simulink model "Pioneer_sim_ucla_mae154S_post"  (Simulink 8.5)
settings: Solver=ode45  StartTime=0.0  StopTime=10000  RelTol=1e-3
model workspace (MATLAB code in the model file):
  | init_dynamics;
values from neighbouring files (symbols this model uses):
  bw = 16.90    (= 16.9)    [get_coeffs.m]    (also in get_coeffs_from_optimization.m; init_dynamics.m)
  cbar = 1.80    (= 1.8)    [get_coeffs.m]    (also in get_coeffs_from_optimization.m; init_dynamics.m)
  grav = 32.17405    [aero_dyn.m]    (also in init_dynamics.m)
  rho = 0.002379    [init_dynamics.m]
  Sw = 30.42    [init_dynamics.m]
  thrust_bx = 89.8    [init_dynamics.m]
libraries: simulink x3
settings Model: Creator=jwm26790  LastModifiedBy=matsuka
settings OptimizationCC: InitFltsAndDblsToZero=on
settings DebuggingCC: SaveWithParameterizedLinksMsg=none  SolverPrmCheckMsg=warning  FcnCallInpInsideContextMsg=UseLocalSettings
settings GRTTargetCC: TargetFcnLib=ansi_tfl_tmw.mat

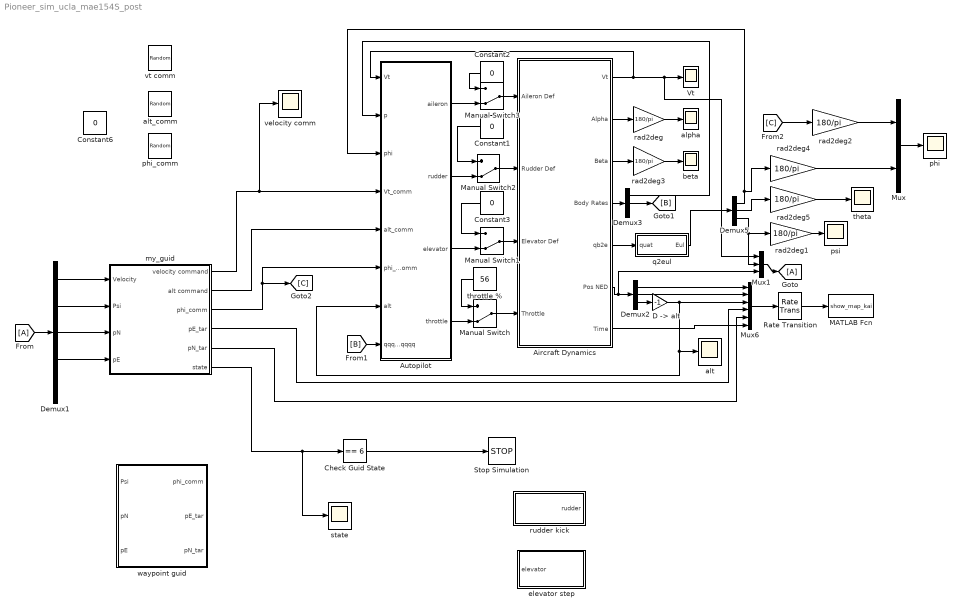
== system Pioneer_sim_ucla_mae154S_post ==
  Aircraft Dynamics : Subsystem
  Autopilot : Subsystem
  Check Guid State : simulink/Logic and Bit Operations/Compare To Constant  relop===  const=6  OutDataTypeStr=boolean
  Constant{1..3,6} (4 alike) : Constant  Value=0
  "D -> alt" : Gain  Gain=-1
  Demux1 : Demux  Outputs=5
  Demux2 : Demux  Outputs=3
  Demux3 : Demux  Outputs=3
  Demux5 : Demux  Outputs=3
  MATLAB Fcn : MATLABFcn  MATLABFcn=show_map_kai  OutputDimensions=0
  Manual Switch{,1..3} (4 alike) : ManualSwitch  CurrentSetting=0
  Mux : Mux  Inputs=2
  Mux1 : Mux  Inputs=[1 1 3]
  Mux6 : Mux  Inputs=6
  Rate Transition : RateTransition  OutPortSampleTime=10
  Stop Simulation : Stop
  Vt : Scope
      settings: TimeRange=50  YMin=131.75  YMax=132.6  SaveName=ScopeData8
  alpha : Scope
      settings: TimeRange=50  YMin=6.9  YMax=7.9
  alt : Scope
      settings: TimeRange=50  YMin=999.5  YMax=1004.5  SaveName=ScopeData14
  alt_comm : UniformRandomNumber  Minimum=1000  Maximum=1500  Seed=2  SampleTime=50
  beta : Scope
      settings: TimeRange=200  YMin=-4  YMax=3  SaveName=ScopeData4
  elevator step : Subsystem
  my_guid : Subsystem
  phi : Scope
      settings: TimeRange=50  YMin=-30  YMax=40  SaveName=ScopeData7
  phi_comm : UniformRandomNumber  Minimum=-.5  Maximum=.5  Seed=3  SampleTime=20
  psi : Scope
      settings: TimeRange=100  YMin=-172.5  YMax=-130  SaveName=ScopeData9
  q2eul : Subsystem
  rad2deg{,1..5} (6 alike) : Gain  Gain=180/pi
  rudder kick : Subsystem
  state : Scope
      settings: TimeRange=50  YMin=2  YMax=2  SaveName=ScopeData15
  theta : Scope
      settings: TimeRange=50  YMin=5.5  YMax=9
  throttle % : Constant  Value=56
  velocity comm : Scope
      settings: TimeRange=50  YMin=100  YMax=100  SaveName=ScopeData16
  vt comm : UniformRandomNumber  Minimum=100  Maximum=130  Seed=2  SampleTime=20
  waypoint guid : Subsystem
  wires:
  Aircraft Dynamics/5(qb2e) -> q2eul/1(quat)
  Aircraft Dynamics/4(Body Rates) -> Demux3/1
  Aircraft Dynamics/1(Vt) -> Autopilot/1(Vt), Vt/1, Mux1/1
  Aircraft Dynamics/6(Pos NED) -> Demux2/1, Mux1/3
  Demux2/3 -> "D -> alt"/1
  "D -> alt"/1 -> Mux6/3, alt/1, Autopilot/7(alt)
  Aircraft Dynamics/2(Alpha) -> rad2deg/1
  rad2deg/1 -> alpha/1
  Aircraft Dynamics/3(Beta) -> rad2deg3/1
  rad2deg3/1 -> beta/1
  q2eul/1(Eul) -> Demux5/1
  Demux5/1 -> Autopilot/3(phi), rad2deg4/1
  Demux3/1 -> Autopilot/2(p)
  Demux2/1 -> Mux6/1
  Demux2/2 -> Mux6/2
  rad2deg1/1 -> psi/1
  rad2deg4/1 -> Mux/2
  rad2deg5/1 -> theta/1
  Demux5/3 -> rad2deg1/1, Mux1/2
  Demux5/2 -> rad2deg5/1
  my_guid/4(pE_tar) -> Mux6/4
  my_guid/5(pN_tar) -> Mux6/5
  Mux1/1 -> [A]
  [A] -> Demux1/1
  Rate Transition/1 -> MATLAB Fcn/1
  Mux6/1 -> Rate Transition/1
  Manual Switch/1 -> Aircraft Dynamics/4(Throttle)
  Manual Switch1/1 -> Aircraft Dynamics/3(Elevator Def)
  throttle %/1 -> Manual Switch/1
  Autopilot/4(throttle) -> Manual Switch/2
  Autopilot/3(elevator) -> Manual Switch1/2
  Manual Switch2/1 -> Aircraft Dynamics/2(Rudder Def)
  Autopilot/2(rudder) -> Manual Switch2/2
  Manual Switch3/1 -> Aircraft Dynamics/1(Aileron Def)
  Autopilot/1(aileron) -> Manual Switch3/2
  Constant2/1 -> Manual Switch3/1
  my_guid/2(alt command) -> Autopilot/5(alt_comm)
  Constant3/1 -> Manual Switch1/1
  Constant1/1 -> Manual Switch2/1
  Demux3/2 -> [B]
  [B] -> Autopilot/8(qqqqqqqqqqqqqqqqqqqqqqqqqqqqqqqqqqqqqqqqqqqqqqqqqqqqqqqqqqqqqqqqqqqqqqqqqqqqqqqqqqqqqqqqqqqqqq)
  my_guid/3(phi_comm) -> Autopilot/6(phi_comm), [C]
  my_guid/1(velocity command) -> velocity comm/1, Autopilot/4(Vt_comm)
  Aircraft Dynamics/7(Time) -> Mux6/6
  Demux1/2 -> my_guid/2(Psi)
  Demux1/3 -> my_guid/3(pN)
  Demux1/4 -> my_guid/4(pE)
  Demux1/1 -> my_guid/1(Velocity)
  [C] -> rad2deg2/1
  Mux/1 -> phi/1
  rad2deg2/1 -> Mux/1
  my_guid/6(state) -> state/1, Check Guid State/1
  Check Guid State/1 -> Stop Simulation/1

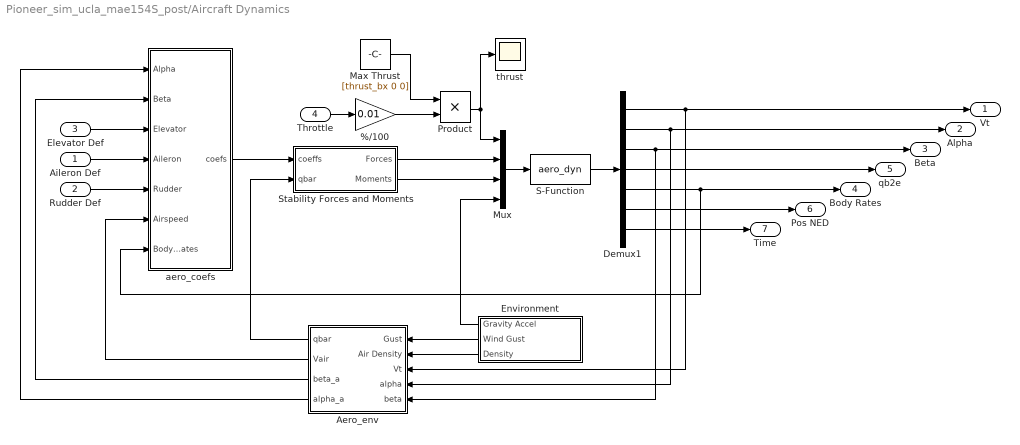
== system Pioneer_sim_ucla_mae154S_post/Aircraft Dynamics ==
  Aileron Def : Inport
  Rudder Def : Inport  Port=2
  Elevator Def : Inport  Port=3
  Throttle : Inport  Port=4
  %/100 : Gain  Gain=0.01
  Aero_env : Subsystem
  Demux1 : Demux  Outputs=[1 1 1 4 3 3 1]
  Environment : Subsystem
  Max Thrust : Constant  Value=[thrust_bx 0 0]
  Mux : Mux
  Product : Product  RndMeth=Zero
  S-Function : S-Function  FunctionName=aero_dyn
  Stability Forces and Moments : Subsystem
  aero_coefs : Subsystem
  thrust : Scope
      settings: YMin=0  YMax=90  SaveName=ScopeData6
  Vt : Outport
  Alpha : Outport  Port=2
  Beta : Outport  Port=3
  Body Rates : Outport  Port=4
  qb2e : Outport  Port=5
  Pos NED : Outport  Port=6
  Time : Outport  Port=7
  wires:
  Demux1/7 -> Time/1
  Demux1/3 -> Aero_env/5(beta), Beta/1
  Demux1/2 -> Aero_env/4(alpha), Alpha/1
  Demux1/1 -> Aero_env/3(Vt), Vt/1
  S-Function/1 -> Demux1/1
  Mux/1 -> S-Function/1
  Demux1/4 -> qb2e/1
  Environment/1(Gravity Accel) -> Mux/4
  Rudder Def/1 -> aero_coefs/5(Rudder)
  Aileron Def/1 -> aero_coefs/4(Aileron)
  Demux1/6 -> Pos NED/1
  Demux1/5 -> aero_coefs/7(Body Rates), Body Rates/1
  Aero_env/2(Vair) -> aero_coefs/6(Airspeed)
  Aero_env/1(qbar) -> Stability Forces and Moments/2(qbar)
  Aero_env/3(beta_a) -> aero_coefs/2(Beta)
  Aero_env/4(alpha_a) -> aero_coefs/1(Alpha)
  Environment/2(Wind Gust) -> Aero_env/1(Gust)
  Environment/3(Density) -> Aero_env/2(Air Density)
  Stability Forces and Moments/1(Forces) -> Mux/2
  aero_coefs/1(coefs) -> Stability Forces and Moments/1(coeffs)
  Stability Forces and Moments/2(Moments) -> Mux/3
  Elevator Def/1 -> aero_coefs/3(Elevator)
  Product/1 -> Mux/1, thrust/1
  Max Thrust/1 -> Product/1
  Throttle/1 -> %/100/1
  %/100/1 -> Product/2

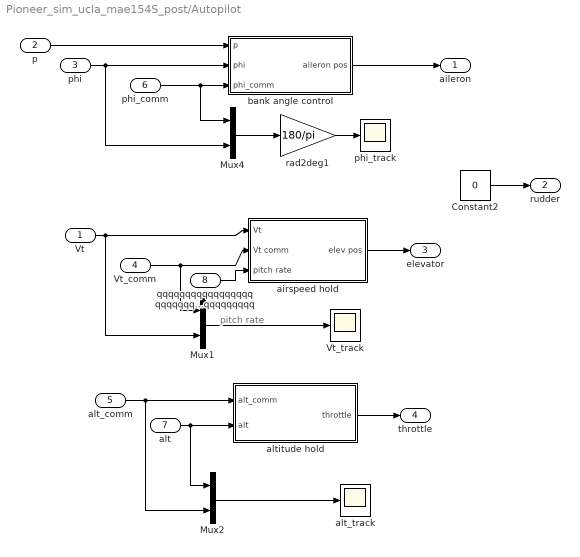
== system Pioneer_sim_ucla_mae154S_post/Autopilot ==
  note: pitch rate
  Vt : Inport
  p : Inport  Port=2
  phi : Inport  Port=3
  Vt_comm : Inport  Port=4
  alt_comm : Inport  Port=5
  phi_comm : Inport  Port=6
  alt : Inport  Port=7
  qqqqqqqqqqqqqqqqqqqqqqqqqqqqqqqqqqqqqqqqqqqqqqqqqqqqqqqqqqqqqqqqqqqqqqqqqqqqqqqqqqqqqqqqqqqqqq : Inport  Port=8
  Constant2 : Constant  Value=0
  Mux1 : Mux  Inputs=2
  Mux2 : Mux  Inputs=2
  Mux4 : Mux  Inputs=2
  Vt_track : Scope
      settings: TimeRange=60  YMin=90  YMax=135  SaveName=ScopeData11
  airspeed hold : Subsystem
  alt_track : Scope
      settings: TimeRange=200  YMin=900  YMax=1600  SaveName=ScopeData12
  altitude hold : Subsystem
  bank angle control : Subsystem
  phi_track : Scope
      settings: TimeRange=200  YMin=-35  YMax=35  SaveName=ScopeData5
  rad2deg1 : Gain  Gain=180/pi
  aileron : Outport
  rudder : Outport  Port=2
  elevator : Outport  Port=3
  throttle : Outport  Port=4
  wires:
  altitude hold/1(throttle) -> throttle/1
  airspeed hold/1(elev pos) -> elevator/1
  bank angle control/1(aileron pos) -> aileron/1
  p/1 -> bank angle control/1(p)
  phi/1 -> bank angle control/2(phi), Mux4/2
  Vt/1 -> airspeed hold/1(Vt), Mux1/2
  alt/1 -> altitude hold/2(alt), Mux2/1
  Mux4/1 -> rad2deg1/1
  rad2deg1/1 -> phi_track/1
  Mux1/1 -> Vt_track/1
  Mux2/1 -> alt_track/1
  alt_comm/1 -> altitude hold/1(alt_comm), Mux2/2
  Vt_comm/1 -> airspeed hold/2(Vt comm), Mux1/1
  phi_comm/1 -> bank angle control/3(phi_comm), Mux4/1
  Constant2/1 -> rudder/1
  qqqqqqqqqqqqqqqqqqqqqqqqqqqqqqqqqqqqqqqqqqqqqqqqqqqqqqqqqqqqqqqqqqqqqqqqqqqqqqqqqqqqqqqqqqqqqq/1 -> airspeed hold/3(pitch rate)

== system Pioneer_sim_ucla_mae154S_post/elevator step ==
  Step4 : Step  Time=5  After=-2*pi/180  SampleTime=0
  Step5 : Step  Time=10  After=10*pi/180  SampleTime=0
  Sum1 : Sum  SaturateOnIntegerOverflow=on
  actuator lag : TransferFcn  Numerator=[10]  Denominator=[1 10]
  elevator1 : Scope
      settings: TimeRange=50  YMin=0  YMax=12  SaveName=ScopeData13
  rad2deg2 : Gain  Gain=180/pi
  elevator : Outport
  wires:
  Step4/1 -> Sum1/1
  rad2deg2/1 -> elevator1/1
  actuator lag/1 -> elevator/1, rad2deg2/1
  Sum1/1 -> actuator lag/1

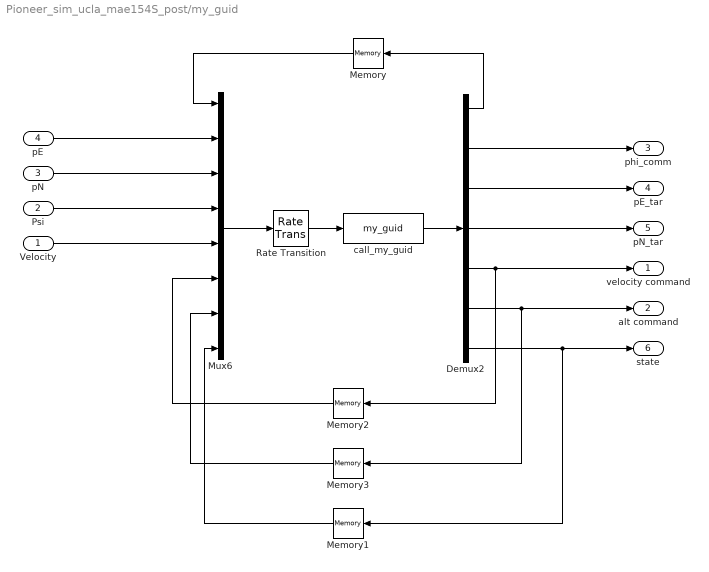
== system Pioneer_sim_ucla_mae154S_post/my_guid ==
  Velocity : Inport
  Psi : Inport  Port=2
  pN : Inport  Port=3
  pE : Inport  Port=4
  Demux2 : Demux  Outputs=7
  Memory : Memory  X0=1
  Memory1 : Memory
  Memory2 : Memory  X0=118.1
  Memory3 : Memory  X0=100
  Mux6 : Mux  Inputs=8
  Rate Transition : RateTransition  OutPortSampleTime=0.1
  call_my_guid : MATLABFcn  MATLABFcn=my_guid  OutputDimensions=7  SampleTime=.5
  velocity command : Outport
  alt command : Outport  Port=2
  phi_comm : Outport  Port=3
  pE_tar : Outport  Port=4
  pN_tar : Outport  Port=5
  state : Outport  Port=6
  wires:
  call_my_guid/1 -> Demux2/1
  Demux2/2 -> phi_comm/1
  Demux2/3 -> pE_tar/1
  Demux2/4 -> pN_tar/1
  pE/1 -> Mux6/2
  pN/1 -> Mux6/3
  Psi/1 -> Mux6/4
  Memory/1 -> Mux6/1
  Rate Transition/1 -> call_my_guid/1
  Mux6/1 -> Rate Transition/1
  Demux2/1 -> Memory/1
  Velocity/1 -> Mux6/5
  Demux2/5 -> Memory2/1, velocity command/1
  Memory1/1 -> Mux6/8
  Memory2/1 -> Mux6/6
  Demux2/7 -> Memory1/1, state/1
  Demux2/6 -> Memory3/1, alt command/1
  Memory3/1 -> Mux6/7

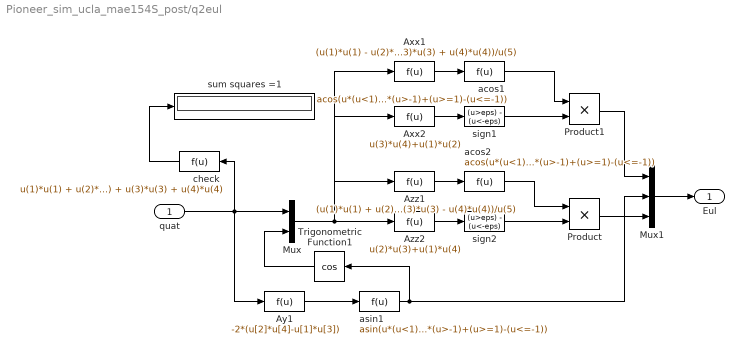
== system Pioneer_sim_ucla_mae154S_post/q2eul ==
  quat : Inport
  Axx1 : Fcn  Expr=(u(1)*u(1) - u(2)*u(2) - u(3)*u(3) + u(4)*u(4))/u(5)
  Axx2 : Fcn  Expr=u(3)*u(4)+u(1)*u(2)
  Ay1 : Fcn  Expr=-2*(u[2]*u[4]-u[1]*u[3])
  Azz1 : Fcn  Expr=(u(1)*u(1) + u(2)*u(2) - u(3)*u(3) - u(4)*u(4))/u(5)
  Azz2 : Fcn  Expr=u(2)*u(3)+u(1)*u(4)
  Mux : Mux  Inputs=2
  Mux1 : Mux  Inputs=3
  Product : Product  SaturateOnIntegerOverflow=on  RndMeth=Zero  InputSameDT=on  OutDataTypeStr=Inherit: Same as first input
  Product1 : Product  SaturateOnIntegerOverflow=on  RndMeth=Zero  InputSameDT=on  OutDataTypeStr=Inherit: Same as first input
  Trigonometric Function1 : Trigonometry  Operator=cos
  acos1 : Fcn  Expr=acos(u*(u<1)*(u>-1)+(u>=1)-(u<=-1))
  acos2 : Fcn  Expr=acos(u*(u<1)*(u>-1)+(u>=1)-(u<=-1))
  "asin1 " : Fcn  Expr=asin(u*(u<1)*(u>-1)+(u>=1)-(u<=-1))
  check : Fcn  Expr=u(1)*u(1) + u(2)*u(2) + u(3)*u(3) + u(4)*u(4)
  sign1 : Fcn  Expr=(u>eps) - (u<-eps)
  sign2 : Fcn  Expr=(u>eps) - (u<-eps)
  sum squares =1 : Display
      settings: Format=long_e
  Eul : Outport  InitialOutput=0
  wires:
  sign1/1 -> Product1/2
  Mux/1 -> Azz2/1, Axx2/1, Azz1/1, Axx1/1
  Trigonometric Function1/1 -> Mux/2
  Ay1/1 -> "asin1 "/1
  Product/1 -> Mux1/3
  acos2/1 -> Product/1
  Product1/1 -> Mux1/1
  acos1/1 -> Product1/1
  sign2/1 -> Product/2
  Axx2/1 -> sign1/1
  Azz1/1 -> acos2/1
  Azz2/1 -> sign2/1
  Axx1/1 -> acos1/1
  "asin1 "/1 -> Mux1/2, Trigonometric Function1/1
  quat/1 -> Mux/1, check/1, Ay1/1
  check/1 -> sum squares =1/1
  Mux1/1 -> Eul/1

== system Pioneer_sim_ucla_mae154S_post/rudder kick ==
  note: rudder kick
  Step1 : Step  Time=10  After=10*pi/180  SampleTime=0
  Step2 : Step  Time=10.5  After=-20*pi/180  SampleTime=0
  Step3 : Step  Time=11  After=10*pi/180  SampleTime=0
  Sum2 : Sum  Inputs=+++  SaturateOnIntegerOverflow=on
  actuator lag : TransferFcn  Numerator=[10]  Denominator=[1 10]
  rad2deg2 : Gain  Gain=180/pi
  rudder1 : Scope
      settings: TimeRange=50  YMin=0  YMax=12  SaveName=ScopeData2
  rudder : Outport
  wires:
  Step1/1 -> Sum2/1
  Step2/1 -> Sum2/2
  Step3/1 -> Sum2/3
  Sum2/1 -> actuator lag/1
  rad2deg2/1 -> rudder1/1
  actuator lag/1 -> rudder/1, rad2deg2/1

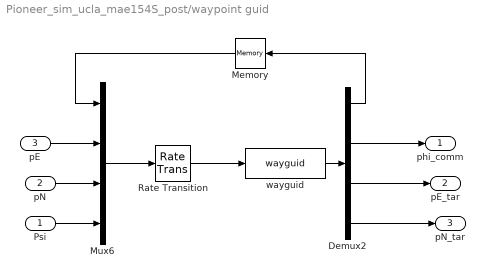
== system Pioneer_sim_ucla_mae154S_post/waypoint guid ==
  Psi : Inport
  pN : Inport  Port=2
  pE : Inport  Port=3
  Demux2 : Demux
  Memory : Memory
  Mux6 : Mux
  Rate Transition : RateTransition  OutPortSampleTime=0.5
  wayguid : MATLABFcn  MATLABFcn=wayguid  OutputDimensions=4  SampleTime=.5
  phi_comm : Outport
  pE_tar : Outport  Port=2
  pN_tar : Outport  Port=3
  wires:
  wayguid/1 -> Demux2/1
  Demux2/2 -> phi_comm/1
  Demux2/3 -> pE_tar/1
  Demux2/4 -> pN_tar/1
  pE/1 -> Mux6/2
  pN/1 -> Mux6/3
  Psi/1 -> Mux6/4
  Memory/1 -> Mux6/1
  Rate Transition/1 -> wayguid/1
  Mux6/1 -> Rate Transition/1
  Demux2/1 -> Memory/1

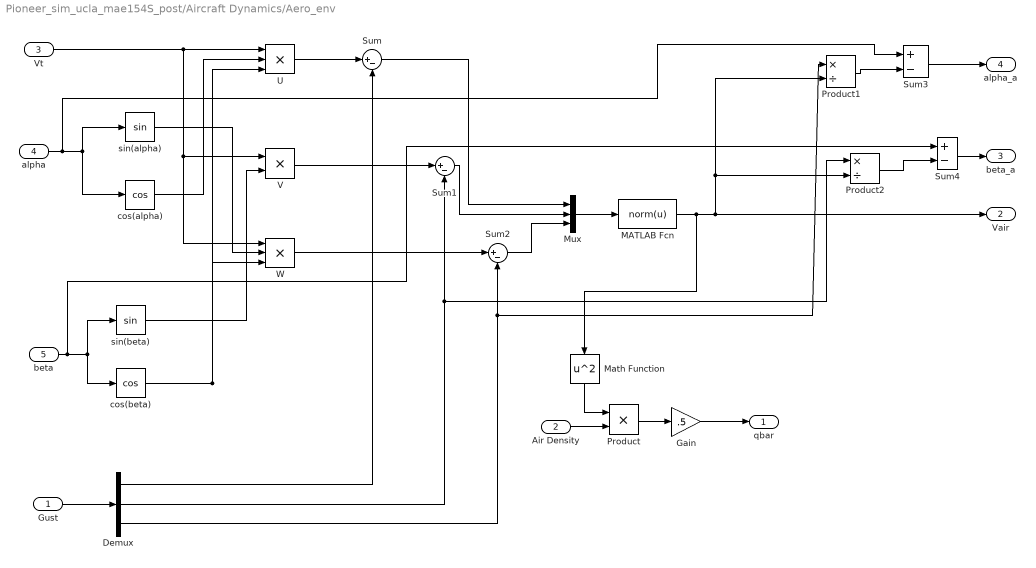
== system Pioneer_sim_ucla_mae154S_post/Aircraft Dynamics/Aero_env ==
  Gust : Inport
  Air Density : Inport  Port=2
  Vt : Inport  Port=3
  alpha : Inport  Port=4
  beta : Inport  Port=5
  Demux : Demux  Outputs=3
  Gain : Gain  Gain=.5
  MATLAB Fcn : MATLABFcn  MATLABFcn=norm(u)
  Math Function : Math  Operator=square  SaturateOnIntegerOverflow=on
  Mux : Mux  Inputs=3
  Product : Product  RndMeth=Zero
  Product1 : Product  Inputs=*/  RndMeth=Zero
  Product2 : Product  Inputs=*/  RndMeth=Zero
  Sum : Sum  Inputs=|+-
  Sum1 : Sum  Inputs=|+-
  Sum2 : Sum  Inputs=|+-
  Sum3 : Sum  Inputs=+-
  Sum4 : Sum  Inputs=+-
  U : Product  Inputs=3
  V : Product
  W : Product  Inputs=3
  cos(alpha) : Trigonometry  Operator=cos
  cos(beta) : Trigonometry  Operator=cos
  sin(alpha) : Trigonometry
  sin(beta) : Trigonometry
  qbar : Outport
  Vair : Outport  Port=2
  beta_a : Outport  Port=3
  alpha_a : Outport  Port=4
  wires:
  alpha/1 -> sin(alpha)/1, cos(alpha)/1, Sum3/1
  beta/1 -> sin(beta)/1, cos(beta)/1, Sum4/1
  Vt/1 -> U/1, V/1, W/1
  cos(alpha)/1 -> U/2
  cos(beta)/1 -> U/3, W/3
  sin(beta)/1 -> V/2
  sin(alpha)/1 -> W/2
  Gust/1 -> Demux/1
  U/1 -> Sum/1
  V/1 -> Sum1/1
  W/1 -> Sum2/1
  Demux/1 -> Sum/2
  Demux/2 -> Sum1/2, Product2/1
  Demux/3 -> Sum2/2, Product1/1
  Mux/1 -> MATLAB Fcn/1
  Sum/1 -> Mux/1
  Sum1/1 -> Mux/2
  Sum2/1 -> Mux/3
  MATLAB Fcn/1 -> Math Function/1, Vair/1, Product1/2, Product2/2
  Math Function/1 -> Product/1
  Air Density/1 -> Product/2
  Product/1 -> Gain/1
  Gain/1 -> qbar/1
  Product1/1 -> Sum3/2
  Sum3/1 -> alpha_a/1
  Product2/1 -> Sum4/2
  Sum4/1 -> beta_a/1

== system Pioneer_sim_ucla_mae154S_post/Aircraft Dynamics/Environment ==
  Constant : Constant  Value=[0; 0; 0]
  Constant Grav : Constant  Value=[0; 0; grav]
  Constant1 : Constant  Value=rho
  Gravity Accel : Outport
  Wind Gust : Outport  Port=2
  Density : Outport  Port=3
  wires:
  Constant/1 -> Wind Gust/1
  Constant1/1 -> Density/1
  Constant Grav/1 -> Gravity Accel/1

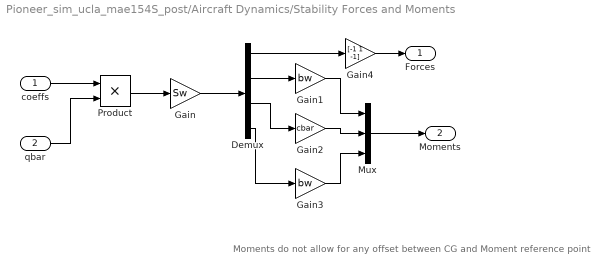
== system Pioneer_sim_ucla_mae154S_post/Aircraft Dynamics/Stability Forces and Moments ==
  note: Moments do not allow for any offset between CG and Moment reference point
  coeffs : Inport
  qbar : Inport  Port=2
  Demux : Demux  Outputs=[3 1 1 1]
  Gain : Gain  Gain=Sw
  Gain1 : Gain  Gain=bw
  Gain2 : Gain  Gain=cbar
  Gain3 : Gain  Gain=bw
  Gain4 : Gain  Gain=[-1 1 -1]
  Mux : Mux  Inputs=3
  Product : Product  RndMeth=Zero
  Forces : Outport
  Moments : Outport  Port=2
  wires:
  coeffs/1 -> Product/1
  qbar/1 -> Product/2
  Product/1 -> Gain/1
  Gain/1 -> Demux/1
  Demux/1 -> Gain4/1
  Demux/2 -> Gain1/1
  Demux/3 -> Gain2/1
  Demux/4 -> Gain3/1
  Gain1/1 -> Mux/1
  Gain2/1 -> Mux/2
  Gain3/1 -> Mux/3
  Mux/1 -> Moments/1
  Gain4/1 -> Forces/1

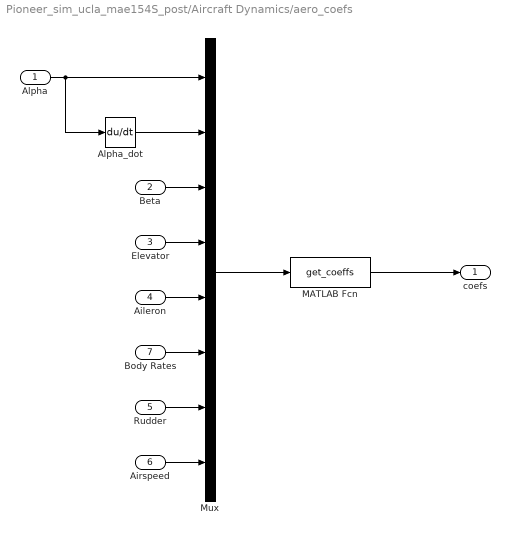
== system Pioneer_sim_ucla_mae154S_post/Aircraft Dynamics/aero_coefs ==
  Alpha : Inport
  Beta : Inport  Port=2
  Elevator : Inport  Port=3
  Aileron : Inport  Port=4
  Rudder : Inport  Port=5
  Airspeed : Inport  Port=6
  Body Rates : Inport  Port=7
  Alpha_dot : Derivative
  MATLAB Fcn : MATLABFcn  MATLABFcn=get_coeffs  OutputDimensions=6
  Mux : Mux  Inputs=[1 1 1 1 1 3 1 1]
  coefs : Outport
  wires:
  Alpha/1 -> Alpha_dot/1, Mux/1
  Alpha_dot/1 -> Mux/2
  Beta/1 -> Mux/3
  Elevator/1 -> Mux/4
  Aileron/1 -> Mux/5
  Rudder/1 -> Mux/7
  Airspeed/1 -> Mux/8
  Mux/1 -> MATLAB Fcn/1
  Body Rates/1 -> Mux/6
  MATLAB Fcn/1 -> coefs/1

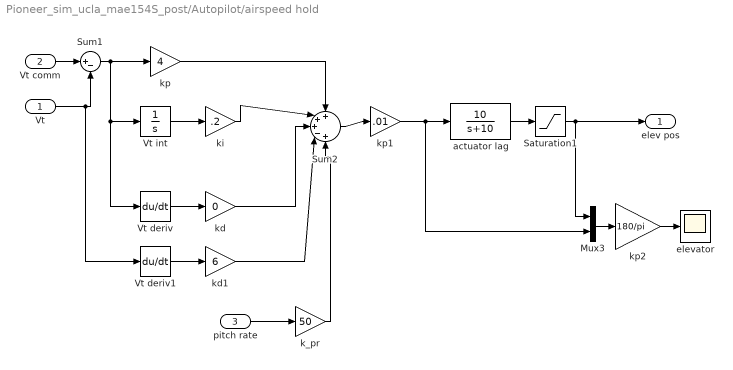
== system Pioneer_sim_ucla_mae154S_post/Autopilot/airspeed hold ==
  Vt : Inport
  Vt comm : Inport  Port=2
  pitch rate : Inport  Port=3
  Mux3 : Mux  Inputs=2
  Saturation1 : Saturate  UpperLimit=15*pi/180  LowerLimit=-15*pi/180
  Sum1 : Sum  Inputs=|+-  SaturateOnIntegerOverflow=on
  Sum2 : Sum  Inputs=+++-+  SaturateOnIntegerOverflow=on
  Vt deriv : Derivative
  Vt deriv1 : Derivative
  Vt int : Integrator
  actuator lag : TransferFcn  Numerator=[10]  Denominator=[1 10]
  elevator : Scope
      settings: TimeRange=60  YMin=-60  YMax=60  SaveName=ScopeData3
  k_pr : Gain  Gain=50
  kd : Gain  Gain=0
  kd1 : Gain  Gain=6
  ki : Gain  Gain=.2
  kp : Gain  Gain=4
  kp1 : Gain  Gain=.01
  kp2 : Gain  Gain=180/pi
  elev pos : Outport
  wires:
  Saturation1/1 -> elev pos/1, Mux3/1
  Sum1/1 -> Vt int/1, Vt deriv/1, kp/1
  kp/1 -> Sum2/1
  Vt int/1 -> ki/1
  Vt deriv/1 -> kd/1
  ki/1 -> Sum2/2
  kd/1 -> Sum2/3
  Sum2/1 -> kp1/1
  kp1/1 -> Mux3/2, actuator lag/1
  Vt comm/1 -> Sum1/1
  Vt/1 -> Sum1/2, Vt deriv1/1
  Vt deriv1/1 -> kd1/1
  kd1/1 -> Sum2/4
  kp2/1 -> elevator/1
  Mux3/1 -> kp2/1
  actuator lag/1 -> Saturation1/1
  pitch rate/1 -> k_pr/1
  k_pr/1 -> Sum2/5

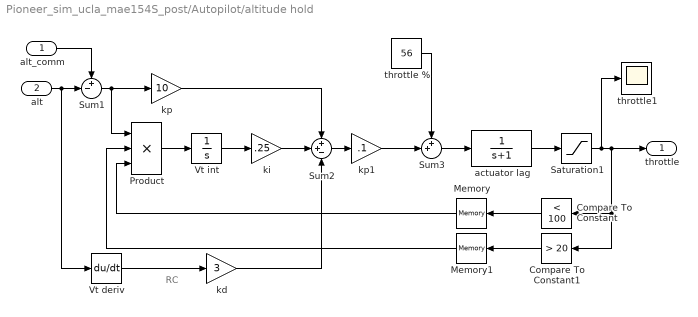
== system Pioneer_sim_ucla_mae154S_post/Autopilot/altitude hold ==
  note: RC
  alt_comm : Inport
  alt : Inport  Port=2
  Compare To Constant : simulink/Logic and Bit Operations/Compare To Constant  relop=<  const=100  OutDataTypeStr=uint8  ZeroCross=off
  Compare To Constant1 : simulink/Logic and Bit Operations/Compare To Constant  relop=>  const=20  OutDataTypeStr=uint8  ZeroCross=off
  Memory : Memory
  Memory1 : Memory
  Product : Product  Inputs=3  RndMeth=Zero
  Saturation1 : Saturate  UpperLimit=100  LowerLimit=20
  Sum1 : Sum  Inputs=+-|  SaturateOnIntegerOverflow=on
  Sum2 : Sum  Inputs=++-  SaturateOnIntegerOverflow=on
  Sum3 : Sum  Inputs=++|  SaturateOnIntegerOverflow=on
  Vt deriv : Derivative
  Vt int : Integrator
  actuator lag : TransferFcn  Denominator=[1 1]
  kd : Gain  Gain=3
  ki : Gain  Gain=.25
  kp : Gain  Gain=10
  kp1 : Gain  Gain=.1
  throttle % : Constant  Value=56
  throttle1 : Scope
      settings: TimeRange=200  YMin=20  YMax=100  SaveName=ScopeData3
  throttle : Outport
  wires:
  alt/1 -> Sum1/2, Vt deriv/1
  alt_comm/1 -> Sum1/1
  actuator lag/1 -> Saturation1/1
  Saturation1/1 -> throttle1/1, throttle/1, Compare To Constant/1, Compare To Constant1/1
  Sum1/1 -> kp/1, Product/1
  kp/1 -> Sum2/1
  Vt int/1 -> ki/1
  Vt deriv/1 -> kd/1
  kd/1 -> Sum2/3
  Sum2/1 -> kp1/1
  throttle %/1 -> Sum3/1
  Sum3/1 -> actuator lag/1
  kp1/1 -> Sum3/2
  ki/1 -> Sum2/2
  Compare To Constant/1 -> Memory/1
  Compare To Constant1/1 -> Memory1/1
  Memory1/1 -> Product/2
  Memory/1 -> Product/3
  Product/1 -> Vt int/1

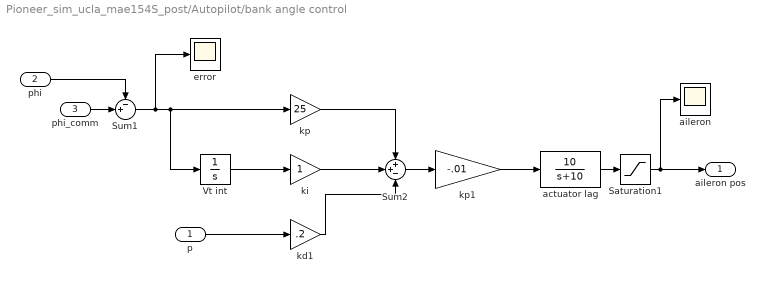
== system Pioneer_sim_ucla_mae154S_post/Autopilot/bank angle control ==
  p : Inport
  phi : Inport  Port=2
  phi_comm : Inport  Port=3
  Saturation1 : Saturate  UpperLimit=.1  LowerLimit=-.1
  Sum1 : Sum  Inputs=-+|  SaturateOnIntegerOverflow=on
  Sum2 : Sum  Inputs=++-  SaturateOnIntegerOverflow=on
  Vt int : Integrator
  actuator lag : TransferFcn  Numerator=[10]  Denominator=[1 10]
  aileron : Scope
      settings: TimeRange=50  YMin=-0.15  YMax=0.09999999999999998  SaveName=ScopeData3
  error : Scope
      settings: TimeRange=50  YMin=-0.15  YMax=0.09999999999999998  SaveName=ScopeData10
  kd1 : Gain  Gain=.2
  ki : Gain
  kp : Gain  Gain=25
  kp1 : Gain  Gain=-.01
  aileron pos : Outport
  wires:
  phi_comm/1 -> Sum1/2
  actuator lag/1 -> Saturation1/1
  Saturation1/1 -> aileron pos/1, aileron/1
  Sum1/1 -> kp/1, Vt int/1, error/1
  kp/1 -> Sum2/1
  Vt int/1 -> ki/1
  ki/1 -> Sum2/2
  Sum2/1 -> kp1/1
  phi/1 -> Sum1/1
  kp1/1 -> actuator lag/1
  kd1/1 -> Sum2/3
  p/1 -> kd1/1
